simulink model "justpulse"  (R2016a)
settings: Solver=VariableStepAuto  StartTime=0.0  StopTime=10  RelTol=1e-3
libraries: simulink x1
settings Model: Creator=Alin anto  LastModifiedBy=Alin anto

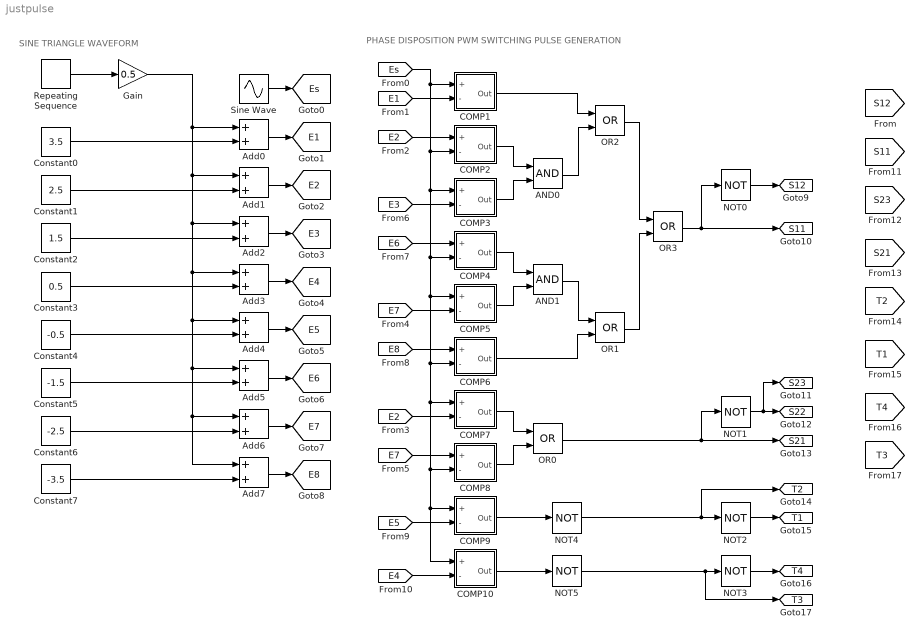
== system justpulse ==
  note: PHASE DISPOSITION PWM SWITCHING PULSE GENERATION
  note: SINE TRIANGLE WAVEFORM
  AND0 : Logic  AllPortsSameDT=off  OutDataTypeStr=boolean
  AND1 : Logic  AllPortsSameDT=off  OutDataTypeStr=boolean
  Add{0..7} (8 alike) : Sum
  COMP1 : Subsystem
  COMP10 : Subsystem
  COMP2 : Subsystem
  COMP3 : Subsystem
  COMP4 : Subsystem
  COMP5 : Subsystem
  COMP6 : Subsystem
  COMP7 : Subsystem
  COMP8 : Subsystem
  COMP9 : Subsystem
  Constant0 : Constant  Value=3.5
  Constant1 : Constant  Value=2.5
  Constant2 : Constant  Value=1.5
  Constant3 : Constant  Value=0.5
  Constant4 : Constant  Value=-0.5
  Constant5 : Constant  Value=-1.5
  Constant6 : Constant  Value=-2.5
  Constant7 : Constant  Value=-3.5
  Gain : Gain  Gain=0.5
  NOT{0..5} (6 alike) : Logic  Operator=NOT  AllPortsSameDT=off  OutDataTypeStr=boolean
  OR{0..3} (4 alike) : Logic  Operator=OR  AllPortsSameDT=off  OutDataTypeStr=boolean
  Repeating Sequence : simulink/Sources/Repeating Sequence  rep_seq_t=[0 5e-5 15e-5 20e-5]  rep_seq_y=[0 1 -1 0]
  Sine Wave : Sin  Amplitude=4  Frequency=2*pi*50  SampleTime=0
  tag scope: E1=global, E2=global, E3=global, E4=global, E5=global, E6=global, E7=global, E8=global, Es=global, S11=global, S12=global, S21=global, S22=global, S23=global, T1=global, T2=global, T3=global, T4=global
  wires:
  COMP1/1(Out) -> OR2/1
  OR0/1 -> [S21], NOT1/1
  OR3/1 -> [S11], NOT0/1
  OR2/1 -> OR3/1
  OR1/1 -> OR3/2
  NOT1/1 -> [S22], [S23]
  NOT0/1 -> [S12]
  COMP4/1(Out) -> AND1/1
  COMP7/1(Out) -> OR0/1
  COMP2/1(Out) -> AND0/1
  COMP6/1(Out) -> OR1/2
  AND0/1 -> OR2/2
  COMP3/1(Out) -> AND0/2
  COMP5/1(Out) -> AND1/2
  AND1/1 -> OR1/1
  COMP8/1(Out) -> OR0/2
  [Es] -> COMP4/2(-), COMP6/2(-), COMP7/1(+), COMP8/2(-), COMP9/1(+), COMP10/1(+), COMP5/1(+), COMP3/1(+), COMP2/2(-), COMP1/1(+)
  [E1] -> COMP1/2(-)
  [E2] -> COMP2/1(+)
  [E3] -> COMP3/2(-)
  [E6] -> COMP4/1(+)
  [E7] -> COMP5/2(-)
  [E8] -> COMP6/1(+)
  [E5] -> COMP9/2(-)
  [E4] -> COMP10/2(-)
  COMP9/1(Out) -> NOT4/1
  NOT4/1 -> [T2], NOT2/1
  NOT2/1 -> [T1]
  COMP10/1(Out) -> NOT5/1
  NOT5/1 -> [T3], NOT3/1
  NOT3/1 -> [T4]
  Constant2/1 -> Add2/2
  Constant3/1 -> Add3/2
  Constant0/1 -> Add0/2
  Constant1/1 -> Add1/2
  Repeating Sequence/1 -> Gain/1
  Gain/1 -> Add7/1, Add6/1, Add5/1, Add4/1, Add3/1, Add2/1, Add1/1, Add0/1
  Constant4/1 -> Add4/2
  Constant6/1 -> Add6/2
  Constant7/1 -> Add7/2
  Constant5/1 -> Add5/2
  Sine Wave/1 -> [Es]
  Add0/1 -> [E1]
  Add1/1 -> [E2]
  Add2/1 -> [E3]
  Add7/1 -> [E8]
  Add6/1 -> [E7]
  Add5/1 -> [E6]
  Add4/1 -> [E5]
  Add3/1 -> [E4]
  [E2] -> COMP7/2(-)
  [E7] -> COMP8/1(+)

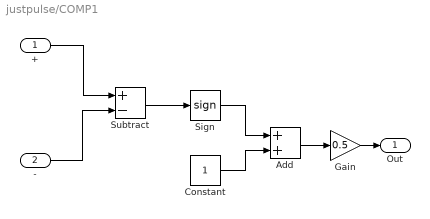
== system justpulse/COMP1 ==
  + : Inport
  - : Inport  Port=2
  Add : Sum
  Constant : Constant
  Gain : Gain  Gain=0.5
  Sign : Signum
  Subtract : Sum  Inputs=+-
  Out : Outport
  wires:
  Add/1 -> Gain/1
  -/1 -> Subtract/2
  Gain/1 -> Out/1
  +/1 -> Subtract/1
  Constant/1 -> Add/2
  Sign/1 -> Add/1
  Subtract/1 -> Sign/1

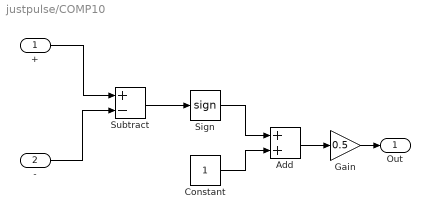
== system justpulse/COMP10 ==
  + : Inport
  - : Inport  Port=2
  Add : Sum
  Constant : Constant
  Gain : Gain  Gain=0.5
  Sign : Signum
  Subtract : Sum  Inputs=+-
  Out : Outport
  wires:
  Add/1 -> Gain/1
  -/1 -> Subtract/2
  Gain/1 -> Out/1
  +/1 -> Subtract/1
  Constant/1 -> Add/2
  Sign/1 -> Add/1
  Subtract/1 -> Sign/1

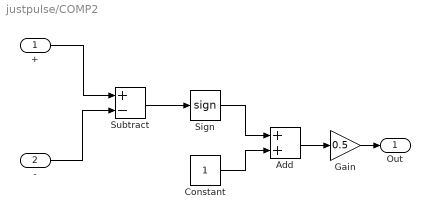
== system justpulse/COMP2 ==
  + : Inport
  - : Inport  Port=2
  Add : Sum
  Constant : Constant
  Gain : Gain  Gain=0.5
  Sign : Signum
  Subtract : Sum  Inputs=+-
  Out : Outport
  wires:
  Add/1 -> Gain/1
  -/1 -> Subtract/2
  Gain/1 -> Out/1
  +/1 -> Subtract/1
  Constant/1 -> Add/2
  Sign/1 -> Add/1
  Subtract/1 -> Sign/1

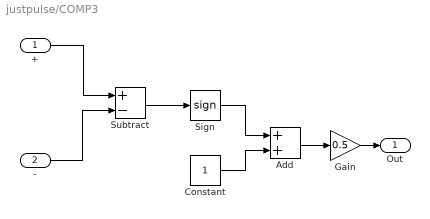
== system justpulse/COMP3 ==
  + : Inport
  - : Inport  Port=2
  Add : Sum
  Constant : Constant
  Gain : Gain  Gain=0.5
  Sign : Signum
  Subtract : Sum  Inputs=+-
  Out : Outport
  wires:
  Add/1 -> Gain/1
  -/1 -> Subtract/2
  Gain/1 -> Out/1
  +/1 -> Subtract/1
  Constant/1 -> Add/2
  Sign/1 -> Add/1
  Subtract/1 -> Sign/1

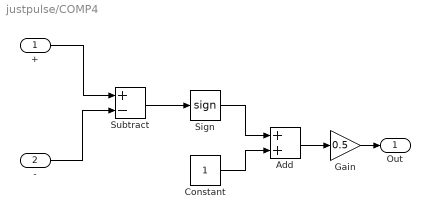
== system justpulse/COMP4 ==
  + : Inport
  - : Inport  Port=2
  Add : Sum
  Constant : Constant
  Gain : Gain  Gain=0.5
  Sign : Signum
  Subtract : Sum  Inputs=+-
  Out : Outport
  wires:
  Add/1 -> Gain/1
  -/1 -> Subtract/2
  Gain/1 -> Out/1
  +/1 -> Subtract/1
  Constant/1 -> Add/2
  Sign/1 -> Add/1
  Subtract/1 -> Sign/1

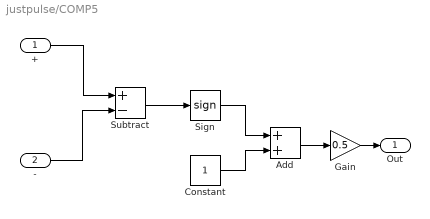
== system justpulse/COMP5 ==
  + : Inport
  - : Inport  Port=2
  Add : Sum
  Constant : Constant
  Gain : Gain  Gain=0.5
  Sign : Signum
  Subtract : Sum  Inputs=+-
  Out : Outport
  wires:
  Add/1 -> Gain/1
  -/1 -> Subtract/2
  Gain/1 -> Out/1
  +/1 -> Subtract/1
  Constant/1 -> Add/2
  Sign/1 -> Add/1
  Subtract/1 -> Sign/1

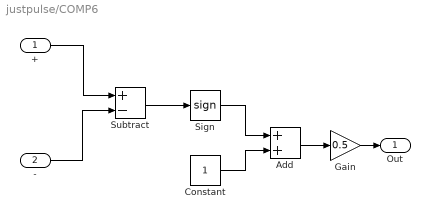
== system justpulse/COMP6 ==
  + : Inport
  - : Inport  Port=2
  Add : Sum
  Constant : Constant
  Gain : Gain  Gain=0.5
  Sign : Signum
  Subtract : Sum  Inputs=+-
  Out : Outport
  wires:
  Add/1 -> Gain/1
  -/1 -> Subtract/2
  Gain/1 -> Out/1
  +/1 -> Subtract/1
  Constant/1 -> Add/2
  Sign/1 -> Add/1
  Subtract/1 -> Sign/1

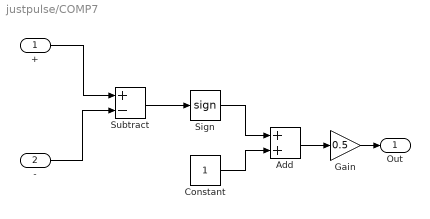
== system justpulse/COMP7 ==
  + : Inport
  - : Inport  Port=2
  Add : Sum
  Constant : Constant
  Gain : Gain  Gain=0.5
  Sign : Signum
  Subtract : Sum  Inputs=+-
  Out : Outport
  wires:
  Add/1 -> Gain/1
  -/1 -> Subtract/2
  Gain/1 -> Out/1
  +/1 -> Subtract/1
  Constant/1 -> Add/2
  Sign/1 -> Add/1
  Subtract/1 -> Sign/1

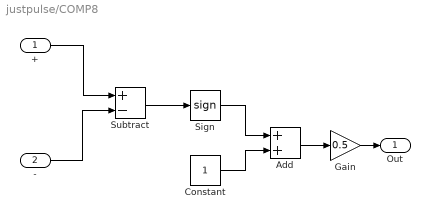
== system justpulse/COMP8 ==
  + : Inport
  - : Inport  Port=2
  Add : Sum
  Constant : Constant
  Gain : Gain  Gain=0.5
  Sign : Signum
  Subtract : Sum  Inputs=+-
  Out : Outport
  wires:
  Add/1 -> Gain/1
  -/1 -> Subtract/2
  Gain/1 -> Out/1
  +/1 -> Subtract/1
  Constant/1 -> Add/2
  Sign/1 -> Add/1
  Subtract/1 -> Sign/1

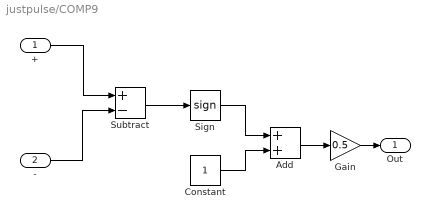
== system justpulse/COMP9 ==
  + : Inport
  - : Inport  Port=2
  Add : Sum
  Constant : Constant
  Gain : Gain  Gain=0.5
  Sign : Signum
  Subtract : Sum  Inputs=+-
  Out : Outport
  wires:
  Add/1 -> Gain/1
  -/1 -> Subtract/2
  Gain/1 -> Out/1
  +/1 -> Subtract/1
  Constant/1 -> Add/2
  Sign/1 -> Add/1
  Subtract/1 -> Sign/1
